simulink model "inertialDynamics"  (R2024a)
settings: configuration reference "standardSILConfiguraitonParams" (kept outside this file)
libraries: shared6dof x1
settings Model: Creator=GTAR  LastModifiedBy=jerem
settings ConfigSetRef: SourceName=standardSILConfiguraitonParams  SourceLocation=Base Workspace

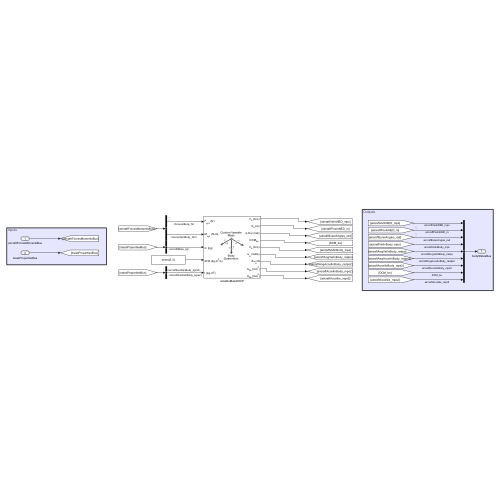
[thumbnail: Simulink's stored preview of the top-level diagram]
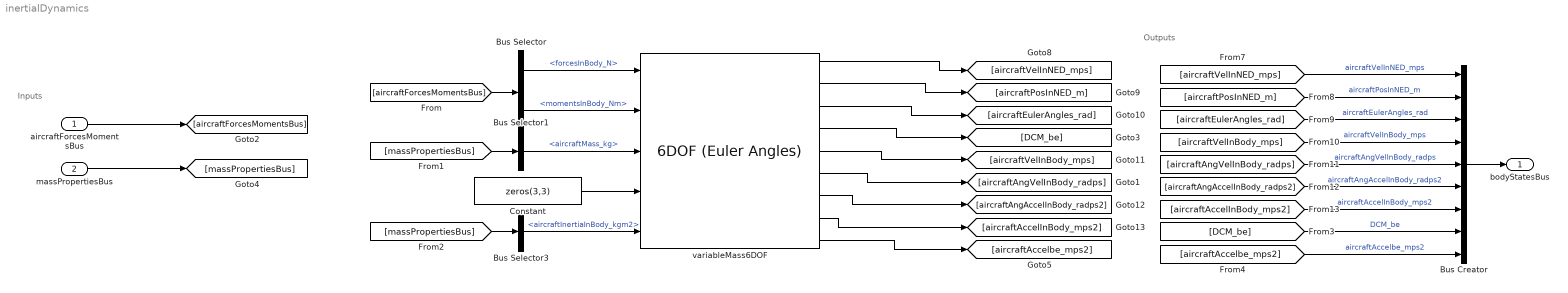
== system inertialDynamics ==
  note: Outputs
  note: Inputs
  aircraftForcesMomentsBus : Inport  OutDataTypeStr=Bus: AircraftForcesMomentsBus
  massPropertiesBus : Inport  Port=2  OutDataTypeStr=Bus: MassPropertiesBus
  Bus Creator : BusCreator  Inputs=9
  Bus Selector : BusSelector  OutputSignals=forcesInBody_N,momentsInBody_Nm
  Bus Selector1 : BusSelector  OutputSignals=aircraftMass_kg
  Bus Selector3 : BusSelector  OutputSignals=aircraftInertiaInBody_kgm2
  Constant : Constant  Value=zeros(3,3)
  variableMass6DOF : shared6dof/6DOF (Euler Angles)  units=Metric (MKS)  mtype=Custom Variable  rep=Quaternion  xme_0=aircraftInitialPosInNED_m  Vm_0=aircraftInitialVelInBody_mps  eul_0=aircraftInitialEuler_rad  pm_0=aircraftInitialBodyRates_radps  mass_0=1.0  mass_e=0.5  mass_f=2.0  inertia=eye(3)  inertia_e=eye(3)  inertia_f=2*eye(3)  k_quat=1.0  vre_flag=off  abi_flag=on  aMode=0  xme_statename=''  Vm_statename=''  eul_statename=''  quat_statename=''  pm_statename=''  mass_statename=''
  bodyStatesBus : Outport  OutDataTypeStr=Bus: BodyStateBus
  wires:
  aircraftForcesMomentsBus/1 -> [aircraftForcesMomentsBus]
  massPropertiesBus/1 -> [massPropertiesBus]
  Bus Selector1/1 -> variableMass6DOF/3  "<aircraftMass_kg>"
  Bus Selector/1 -> variableMass6DOF/1  "<forcesInBody_N>"
  Constant/1 -> variableMass6DOF/4
  [aircraftVelInNED_mps] -> Bus Creator/1  "aircraftVelInNED_mps"
  [aircraftAccelInBody_mps2] -> Bus Creator/7  "aircraftAccelInBody_mps2"
  [aircraftVelInBody_mps] -> Bus Creator/4  "aircraftVelInBody_mps"
  [aircraftAngVelInBody_radps] -> Bus Creator/5  "aircraftAngVelInBody_radps"
  [aircraftEulerAngles_rad] -> Bus Creator/3  "aircraftEulerAngles_rad"
  [aircraftPosInNED_m] -> Bus Creator/2  "aircraftPosInNED_m"
  Bus Selector/2 -> variableMass6DOF/2  "<momentsInBody_Nm>"
  [aircraftForcesMomentsBus] -> Bus Selector/1
  [massPropertiesBus] -> Bus Selector1/1
  [massPropertiesBus] -> Bus Selector3/1
  Bus Selector3/1 -> variableMass6DOF/5  "<aircraftInertiaInBody_kgm2>"
  Bus Creator/1 -> bodyStatesBus/1
  [aircraftAngAccelInBody_radps2] -> Bus Creator/6  "aircraftAngAccelInBody_radps2"
  [DCM_be] -> Bus Creator/8  "DCM_be"
  variableMass6DOF/1 -> [aircraftVelInNED_mps]
  variableMass6DOF/8 -> [aircraftAccelInBody_mps2]
  variableMass6DOF/7 -> [aircraftAngAccelInBody_radps2]
  variableMass6DOF/6 -> [aircraftAngVelInBody_radps]
  variableMass6DOF/5 -> [aircraftVelInBody_mps]
  variableMass6DOF/4 -> [DCM_be]
  variableMass6DOF/3 -> [aircraftEulerAngles_rad]
  variableMass6DOF/2 -> [aircraftPosInNED_m]
  variableMass6DOF/9 -> [aircraftAccelbe_mps2]
  [aircraftAccelbe_mps2] -> Bus Creator/9  "aircraftAccelbe_mps2"
